simulink model "ad_des_sim6"  (R2023a)
settings: Solver=ode15s  StartTime=0.0  StopTime=simulation_time  MaxStep=20
model workspace (MAT data in the model file):
  adsorpQ = SimulinkDemos.Signal
  adsorpQ.DataType = 'auto'
  adsorpQ.Dimensions = -1
  adsorpQ.DimensionsMode = 'auto'
  adsorpQ.Complexity = 'auto'
  adsorpQ.SampleTime = -1
  adsorpQ.SamplingMode = 'auto'
values from neighbouring files (symbols this model uses):
  Adsorption_time = 70    [run_this_file.m]
  Desorption_time = 20    [run_this_file.m]
  Rinsing_time = 10    [run_this_file.m]
  standby_time = abs(Adsorption_time-(Desorption_time+Rinsing_time))    [run_this_file.m]
libraries: dspsigops x1
settings Model: Creator=saasa  LastModifiedBy=ASUSTEK
settings SolverCC: AlgebraicLoopSolver=TrustRegion
settings DataIOCC: SaveFinalState=on  SaveState=on
settings DebuggingCC: UnconnectedInputMsg=warning  UnconnectedOutputMsg=warning  UnconnectedLineMsg=warning
settings ModelReferenceCC: EnableRefExpFcnMdlSchedulingChecks=on

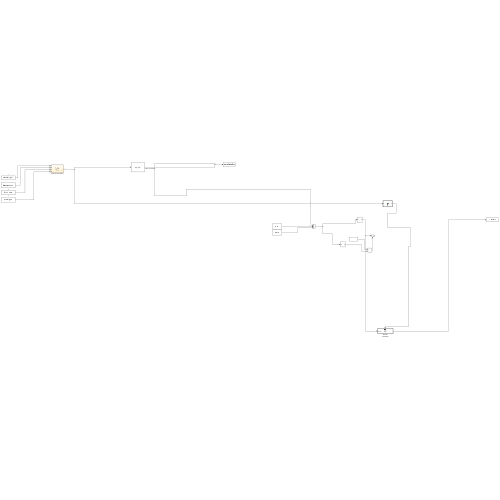
[thumbnail: Simulink's stored preview of the top-level diagram]
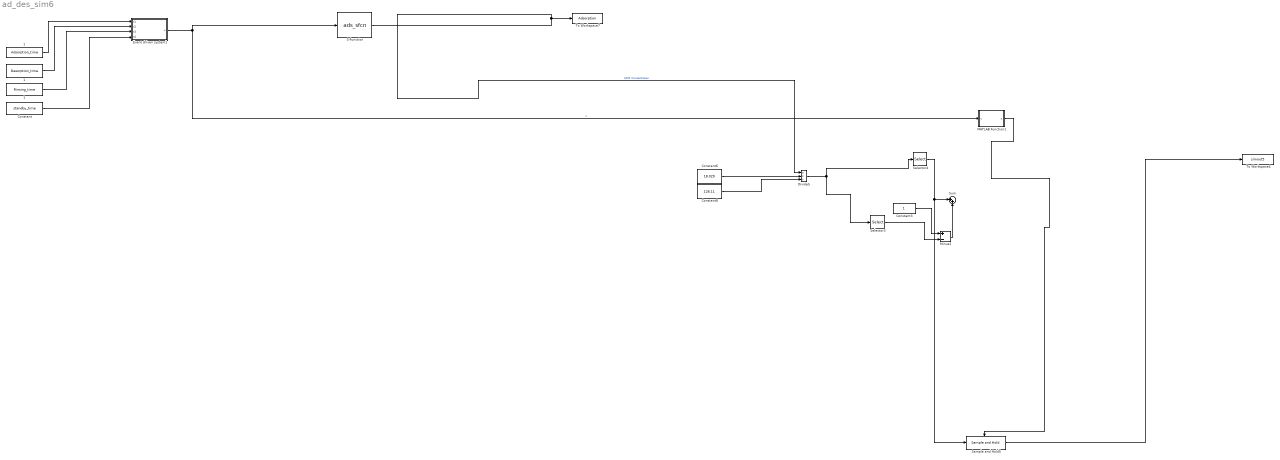
== system ad_des_sim6 ==
  "   1" : Constant  Value=Adsorption_time
  "  1" : Constant  Value=Desorption_time
  " 1" : Constant  Value=Rinsing_time
  Constant : Constant  Value=standby_time
  Constant3 : Constant
  Constant6 : Constant  Value=18.029
  Constant8 : Constant  Value=126.11
  Divide5 : Product  Inputs=**/
  Event driven system1 : Stateflow chart  TreatAsAtomicUnit=on
  MATLAB Function1 : MATLAB Function  TreatAsAtomicUnit=on
  Minus2 : Sum  Inputs=+-
  S-Function : S-Function  FunctionName=ads_sfcn  SFunctionDeploymentMode=off  EnableBusSupport=off
  Sample and Hold5 : dspsigops/Sample and Hold  trig=Falling edge  initCond=0  latchinput=on
  Selector3 : Selector  InputPortWidth=110  IndexOptions=Index vector (dialog)  Indices=55  OutputSizes=1
  Selector4 : Selector  InputPortWidth=110  IndexOptions=Index vector (dialog)  Indices=55  OutputSizes=1
  Sum : Sum  Inputs=|++
  To Workspace4 : ToWorkspace  VariableName=simout5  SaveFormat=Timeseries  SampleTime=-1
  To Workspace7 : ToWorkspace  VariableName=Adsorption  SaveFormat=Timeseries  SampleTime=-1
  wires:
  S-Function/1 -> To Workspace7/1, Divide5/1  "HMF Concentraion"
  " 1"/1 -> Event driven system1/3(t3)
  "   1"/1 -> Event driven system1/1(t1)
  Constant3/1 -> Minus2/1
  Minus2/1 -> Sum/2
  Event driven system1/1(u) -> S-Function/1, MATLAB Function1/1(u)  "u"
  Constant/1 -> Event driven system1/4(t4)
  "  1"/1 -> Event driven system1/2(t2)
  MATLAB Function1/1(y) -> Sample and Hold5/Trigger
  Constant6/1 -> Divide5/2
  Constant8/1 -> Divide5/3
  Divide5/1 -> Selector3/1, Selector4/1
  Selector4/1 -> Sample and Hold5/1, Sum/1
  Selector3/1 -> Minus2/2
  Sample and Hold5/1 -> To Workspace4/1

== stateflow chart ad_des_sim6/Event driven system1 ==
  settings: updateMethod=CONTINUOUS
  state ADS0
    ex:
    du,en: u = 1;
  state ADS
    ex:
    du,en: u = 1;
  state DEP
    ex:
    du,en: u = 2;
  state BDN
    ex:
    du,en: u = 3;
  state PRG
    ex:
    du,en: u = 4;
  (default) -> ADS0
  ADS0 -> DEP : [after(t1,sec)]
  PRG -> ADS : [after(t4,sec)]
  ADS -> DEP : [after(t1,sec)]
  DEP -> BDN : [after(t2,sec)]
  BDN -> PRG : [after(t3,sec)]
  data: t1 input double; t2 input double; t3 input double; t4 input double; u output

== matlab function ad_des_sim6/MATLAB Function1 ==
  data: u input; y output
function y = fcn(u)
if u==1
    y=1;
else 
    y=0;
end
end
